simulink model "nlms"  (R2020a)
settings: Solver=VariableStepAuto  StartTime=0.0  StopTime=5  RelTol=1e-3
model workspace (MAT data in the model file):
  constellation = Simulink.DualScaledParameter
  constellation.DataType = 'auto'
  constellation.Dimensions = [0 0]
libraries: dspvision x2, dsparch4 x1, dspadpt3 x1
settings Model: Creator=ASUS  LastModifiedBy=ASUS

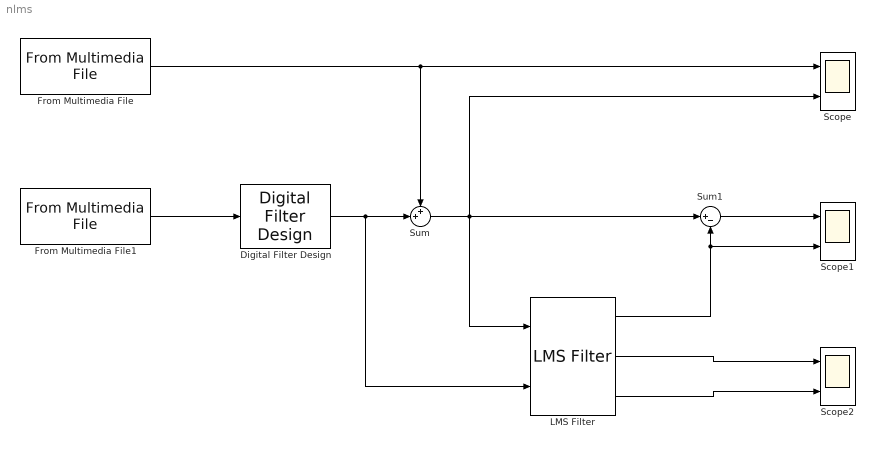
== system nlms ==
  Digital Filter Design : dsparch4/Digital Filter Design  mwdsp_browser_bugfix_var=off
  From Multimedia File : dspvision/From Multimedia File  inputFilename=C:\Program Files\Polyspace\R2020a\toolbox\dsp\dsp\speech_dft.wav  readRange=[1 Inf]  loop=on  numPlays=inf  outputStreams=Audio only  videoDataType=single  audioDataType=double  inheritSampleTime=on  userDefinedSampleTime=1/30  noAudioOutput=off  isIntensityVideo=off  fourcc=RGB  colorVideoFormat=Separate color signals  outputEOF=off  dataOrg=Column-major  audioFrameSize=1024  computeAudioFrameSize=off  outSamplingMode=Sample based
  From Multimedia File1 : dspvision/From Multimedia File  inputFilename=C:\Program Files\Polyspace\R2020a\toolbox\dsp\dsp\audio48kHz.wav  readRange=[1 Inf]  loop=on  numPlays=inf  outputStreams=Audio only  videoDataType=single  audioDataType=double  inheritSampleTime=on  userDefinedSampleTime=1/30  noAudioOutput=off  isIntensityVideo=off  fourcc=RGB  colorVideoFormat=Separate color signals  outputEOF=off  dataOrg=Column-major  audioFrameSize=1024  computeAudioFrameSize=off  outSamplingMode=Sample based
  LMS Filter : dspadpt3/LMS Filter  Algo=Normalized LMS  L=32  stepflag=Dialog  mu=0.1  leakage=1.0  ic=0  Adapt=off  resetflag=None  weights=on  addnparflag=off  roundingMode=Floor  overflowMode=off
      settings: SourceProductBaseCode=DS
  Scope : Scope  NumInputPorts=2
  Scope1 : Scope  NumInputPorts=2
  Scope2 : Scope  NumInputPorts=2
  Sum : Sum  Inputs=++|
  Sum1 : Sum  Inputs=|+-
  wires:
  From Multimedia File/1 -> Sum/1, Scope/1
  From Multimedia File1/1 -> Digital Filter Design/1
  Digital Filter Design/1 -> Sum/2, LMS Filter/2
  Sum/1 -> Sum1/1, LMS Filter/1, Scope/2
  LMS Filter/1 -> Sum1/2, Scope1/2
  Sum1/1 -> Scope1/1
  LMS Filter/2 -> Scope2/1
  LMS Filter/3 -> Scope2/2
